simulink model "MOTHERofALL3"  (Simulink 7.7)
settings: Solver=VariableStepDiscrete  StartTime=0  StopTime=2  RelTol=1e-3
undefined symbols (not defined in the file): Acid, Lead, Ptotal, Qtotal, ts
libraries: powerlib x20, powerlib_extras x7, simulink x5, electricdrivelib x1
settings Model: Creator=chico  LastModifiedBy=elacpr

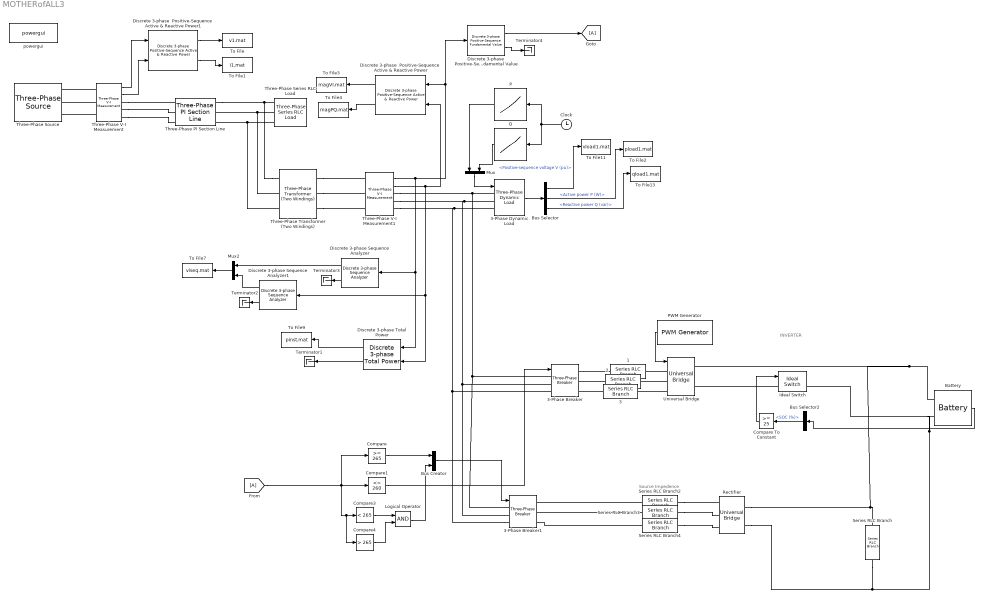
== system MOTHERofALL3 ==
  note: Source Impedence
  note: INVERTER
  1 : powerlib/Elements/Series RLC Branch  PhysicalDomain=powersysdomain  SubClassName=unknown  LeftPortType=p1  RightPortType=p1  LConnTagsString=__new0  RConnTagsString=__new0  BranchType=L  Resistance=1  Inductance=1  SetiL0=off  InitialCurrent=0  Capacitance=1e-6  Setx0=off  InitialVoltage=0  Measurements=None
  2 : powerlib/Elements/Series RLC Branch  PhysicalDomain=powersysdomain  SubClassName=unknown  LeftPortType=p1  RightPortType=p1  LConnTagsString=__new0  RConnTagsString=__new0  BranchType=L  Resistance=1  Inductance=1  SetiL0=off  InitialCurrent=0  Capacitance=1e-6  Setx0=off  InitialVoltage=0  Measurements=None
  3 : powerlib/Elements/Series RLC Branch  PhysicalDomain=powersysdomain  SubClassName=unknown  LeftPortType=p1  RightPortType=p1  LConnTagsString=__new0  RConnTagsString=__new0  BranchType=L  Resistance=1  Inductance=1  SetiL0=off  InitialCurrent=0  Capacitance=1e-6  Setx0=off  InitialVoltage=0  Measurements=None
  3-Phase Dynamic Load : powerlib/Elements/Three-Phase Dynamic Load  SystemSampleTime=-1  NominalVoltage=[ 400 60 ]  ActiveReactivePowers=[50 25]  PositiveSequence=[0.292838 -10.4312]  ExternalControl=on  NpNq="[1  1]"  TimeConstants="[0  0  0  0]"  MinimumVoltage=0.7  LoadFlowParameters=[4 50 0 0 25]
  3-Phase Breaker : powerlib/Elements/Three-Phase Breaker  SystemSampleTime=-1  InitialState=open  SwitchA=on  SwitchB=on  SwitchC=on  SwitchTimes="[4/60  10/60]"  External=on  BreakerResistance=0.001  SnubberResistance=1e6  SnubberCapacitance=inf  Measurements=None
  3-Phase Breaker1 : powerlib/Elements/Three-Phase Breaker  SystemSampleTime=-1  InitialState=open  SwitchA=on  SwitchB=on  SwitchC=on  SwitchTimes="[4/60  10/60]"  External=on  BreakerResistance=0.001  SnubberResistance=1e6  SnubberCapacitance=inf  Measurements=None
  Battery : electricdrivelib/Extra Sources/Battery  SystemSampleTime=-1  BatType=Lead-Acid  ShowDetailedParameters=off  NomV=240  NomQ=10  SOC=80  PresetModel=off  MaxQ=1.6154  FullV=1.4136  Dis_rate=0.3  R=0.008  Normal_OP=1.4423  expZone="[1.3017         0.3]"  Dis_Char=off  current=[1.5 3]  Units=Ampere-hour  Batt_Tr=30
  Bus Creator : BusCreator  Inputs=2
  Bus Selector : BusSelector  OutputSignals=Positive-sequence voltage V (pu),Active power P (W),Reactive power Q (var)
  Bus Selector2 : BusSelector  OutputSignals=SOC (%)
  Clock : Clock
  Compare : simulink/Logic and Bit Operations/Compare To Constant  SystemSampleTime=-1  relop=>=  const=265  LogicOutDataTypeMode=uint8
  Compare To Constant : simulink/Logic and Bit Operations/Compare To Constant  SystemSampleTime=-1  relop=>=  const=25  LogicOutDataTypeMode=uint8
  Compare1 : simulink/Logic and Bit Operations/Compare To Constant  SystemSampleTime=-1  relop=<=  const=260  LogicOutDataTypeMode=uint8
  Compare3 : simulink/Logic and Bit Operations/Compare To Constant  SystemSampleTime=-1  relop=<  const=265  LogicOutDataTypeMode=uint8
  Compare4 : simulink/Logic and Bit Operations/Compare To Constant  SystemSampleTime=-1  relop=>  const=265  LogicOutDataTypeMode=uint8
  Discrete 3-phase Positive-Sequence Fundamental Value : powerlib_extras/Discrete Measurements/Discrete 3-phase Positive-Sequence Fundamental Value  SystemSampleTime=-1  Freq=60  Par_Init=[0 0]  Ts=50e-6
  Discrete 3-phase Sequence Analyzer : powerlib_extras/Discrete Measurements/Discrete 3-phase Sequence Analyzer  SystemSampleTime=-1  Freq=60  n=1  seq=Positive  Par_Init=[0 0]  Ts=50e-6
  Discrete 3-phase Sequence Analyzer1 : powerlib_extras/Discrete Measurements/Discrete 3-phase Sequence Analyzer  SystemSampleTime=-1  Freq=60  n=1  seq=Positive  Par_Init=[0 0]  Ts=50e-6
  Discrete 3-phase Total Power : powerlib_extras/Discrete Measurements/Discrete 3-phase Total Power  SystemSampleTime=-1  Freq=60  Par_Vinit=[0 0]  Par_Iinit=[0 0]  Ts=50e-6
  Discrete 3-phase  Positive-Sequence  Active & Reactive Power : powerlib_extras/Discrete Measurements/Discrete 3-phase  Positive-Sequence  Active & Reactive Power  SystemSampleTime=-1  Freq=60  Par_Vinit=[0 0]  Par_Iinit=[0 0]  Ts=50e-6
  Discrete 3-phase  Positive-Sequence  Active & Reactive Power1 : powerlib_extras/Discrete Measurements/Discrete 3-phase  Positive-Sequence  Active & Reactive Power  SystemSampleTime=-1  Freq=60  Par_Vinit=[0 0]  Par_Iinit=[0 0]  Ts=50e-6
  Ideal Switch : powerlib/Power Electronics/Ideal Switch  SystemSampleTime=-1  Ron=0.001  Lon=0  IC=0  Rs=1e5  Cs=inf  Measurements=on
  Logical Operator : Logic  AllPortsSameDT=off  OutDataTypeStr=boolean
  Mux : Mux  Inputs=2
  Mux2 : Mux  Inputs=2
  P : Lookup  InputValues=ts  Table=Ptotal
  PWM Generator : powerlib_extras/Control  Blocks/PWM Generator  SystemSampleTime=-1  GeneratorMode="3-arm  bridge (6 pulses)"  Fc=1080  Internal=on  mIndex=0.4  Freq=50  Phase=0
  Q : Lookup  InputValues=ts  Table=Qtotal
  Rectifier : powerlib/Power Electronics/Universal Bridge  SystemSampleTime=-1  Arms=3  SnubberResistance=100  SnubberCapacitance=0.1e-6  Device=Diodes  Ron=1e-3  Lon=0  ForwardVoltages="[  0.8  0.8  ]"  ForwardVoltage=.8  GTOparameters=[ 10e-6 , 20e-6 ]  IGBTparameters=[ 1e-6 , 2e-6 ]  Measurements=Device currents  Measurements_2=None  converterType=Rectifier
  Series RLC Branch : powerlib/Elements/Series RLC Branch  PhysicalDomain=powersysdomain  SubClassName=unknown  LeftPortType=p1  RightPortType=p1  LConnTagsString=__new0  RConnTagsString=__new0  BranchType=C  Resistance=5  Inductance=1e-3  SetiL0=off  InitialCurrent=0  Capacitance=470e-6  Setx0=off  InitialVoltage=0  Measurements=None
  Series RLC Branch2 : powerlib/Elements/Series RLC Branch  PhysicalDomain=powersysdomain  SubClassName=unknown  LeftPortType=p1  RightPortType=p1  LConnTagsString=__new0  RConnTagsString=__new0  BranchType=RL  Resistance=0.5  Inductance=1e-3  SetiL0=off  InitialCurrent=0  Capacitance=200e-6  Setx0=off  InitialVoltage=0  Measurements=None
  Series RLC Branch3 : powerlib/Elements/Series RLC Branch  PhysicalDomain=powersysdomain  SubClassName=unknown  LeftPortType=p1  RightPortType=p1  LConnTagsString=__new0  RConnTagsString=__new0  BranchType=RL  Resistance=0.5  Inductance=1e-3  SetiL0=off  InitialCurrent=0  Capacitance=200e-6  Setx0=off  InitialVoltage=0  Measurements=None
  Series RLC Branch4 : powerlib/Elements/Series RLC Branch  PhysicalDomain=powersysdomain  SubClassName=unknown  LeftPortType=p1  RightPortType=p1  LConnTagsString=__new0  RConnTagsString=__new0  BranchType=RL  Resistance=0.5  Inductance=1e-3  SetiL0=off  InitialCurrent=0  Capacitance=200e-6  Setx0=off  InitialVoltage=0  Measurements=None
  Terminator{1..4} (4 alike) : Terminator
  Three-Phase PI Section Line : powerlib/Elements/Three-Phase PI Section Line  PhysicalDomain=powersysdomain  SubClassName=unknown  LeftPortType=p1  RightPortType=p1  LConnTagsString=a|b|c  RConnTagsString=A|B|C  Frequency=60  Resistances=[ 0.01273 0.3864]  Inductances="[ 0.9337e-3  4.1264e-3]"  Capacitances=[12.74e-9 7.751e-9]  Length=10
  Three-Phase Series RLC Load : powerlib/Elements/Three-Phase Series RLC Load  PhysicalDomain=powersysdomain  SubClassName=unknown  LeftPortType=p1  RightPortType=p1  LConnTagsString=A|B|C  Configuration=Y (grounded)  NominalVoltage=13800  NominalFrequency=60  ActivePower=10e6  InductivePower=1000  CapacitivePower=0  Measurements=None  LoadType=constant Z
  Three-Phase Transformer (Two Windings) : powerlib/Elements/Three-Phase Transformer (Two Windings)  SystemSampleTime=-1  Winding1Connection=Yg  UNITS=SI  NominalPower=[ 25e3 , 60 ]  Winding1=[13800 27.648 0.220022]  Winding2Connection=Yg  Winding2=[240 0.00384 0]  SetSaturation=off  Rm=1.3824e5  Lm=366  Saturation=[0 0;6.6653e-005 1910.3;0.027772 2419.7]  Hysteresis=off  DataFile='hysteresis'  SetInitialFlux=off  InitialFluxes=[1273.5 -1273.5 1114.3]  Measurements=None  MoreParameters=off  BreakLoop=off  DataType=on  TransfoNumber=1
  Three-Phase V-I Measurement : powerlib/Measurements/Three-Phase V-I Measurement  SystemSampleTime=-1  VoltageMeasurement=phase-to-ground  SetLabelV=off  LabelV=Vabc  Vpu=off  VpuLL=off  CurrentMeasurement=yes  SetLabelI=off  LabelI=Iabc  Ipu=off  Pbase=100e6  Vbase=500e3  OutputType=Complex  PhasorSimulation=off  PSBequivalent=0
  Three-Phase V-I Measurement1 : powerlib/Measurements/Three-Phase V-I Measurement  SystemSampleTime=-1  VoltageMeasurement=phase-to-phase  SetLabelV=off  LabelV=Vabc  Vpu=off  VpuLL=off  CurrentMeasurement=yes  SetLabelI=off  LabelI=Iabc  Ipu=off  Pbase=100e6  Vbase=240  OutputType=Complex  PhasorSimulation=off  PSBequivalent=0
  Three-Phase Source : powerlib/Electrical Sources/Three-Phase Source  SystemSampleTime=-1  Voltage=13800  PhaseAngle=0  Frequency=60  InternalConnection=Yg  SpecifyImpedance=off  Resistance=0.001  Inductance=0.000001  ShortCircuitLevel=100e6  BaseVoltage=25e3  XRratio=7  BusType=swing  Pref=0  Qref=0  Qmin=-inf  Qmax=inf
  To File : ToFile  Filename=v1.mat  MatrixName=v1
      settings: Decimation=200
  To File1 : ToFile  Filename=i1.mat  MatrixName=i1
      settings: Decimation=200
  To File11 : ToFile  Filename=vload1.mat  MatrixName=vl1
      settings: Decimation=20000
  To File13 : ToFile  Filename=qload1.mat  MatrixName=ql1
      settings: Decimation=20000
  To File2 : ToFile  Filename=pload1.mat  MatrixName=pl1
      settings: Decimation=20000
  To File3 : ToFile  Filename=magVI.mat  MatrixName=vi
      settings: Decimation=20000
  To File4 : ToFile  Filename=magPQ.mat  MatrixName=pq
      settings: Decimation=20000
  To File7 : ToFile  Filename=viseq.mat  MatrixName=viseq
      settings: Decimation=20000
  To File9 : ToFile  Filename=pinst.mat  MatrixName=pinst
      settings: Decimation=200
  Universal Bridge : powerlib/Power Electronics/Universal Bridge  SystemSampleTime=-1  Arms=3  SnubberResistance=1e5  SnubberCapacitance=inf  Device=IGBT / Diodes  Ron=1e-3  Lon=0  ForwardVoltages="[  0  0  ]"  ForwardVoltage=0  GTOparameters=[ 10e-6 , 20e-6 ]  IGBTparameters=[ 1e-6 , 2e-6 ]  Measurements=None  Measurements_2=None  converterType=Rectifier
  powergui : powerlib/powergui  Priority=1  SystemSampleTime=-1  SimulationMode=Discrete  SampleTime=50e-4  frequency=60  SPID=off  DisableSnubberDevices=off  DisableRonSwitches=off  DisableVfSwitches=off  SwTol=0  Interpol=off  DisplayEquations=off  FunctionMessages=off  frequencyindice=60  Pbase=100e6  ErrMax=1e-4  Iterations=50  UnitsV=kV  UnitsW=MW  echomessages=off  HookPort=off  EnableUseOfTLC=off  x0status=blocks  RestoreLinks=warning  ResistiveCurrentMeasurement=off  Ylog=off  Xlog=on  ShowGrid=off  save=off  variable=ZData  ZoomFFT=off  StartTime=0.0  cycles=1  DisplayStyle=1  FreqAxis=off  MaxFrequency=1000  frequencyindicesteady=1  display=off  methode=off
  wires:
  P/1 -> Mux/1
  Q/1 -> Mux/2
  Clock/1 -> Q/1, P/1
  Mux/1 -> 3-Phase Dynamic Load/1
  Three-Phase V-I Measurement1/1 -> Discrete 3-phase Total Power/1, Discrete 3-phase Sequence Analyzer/1, Discrete 3-phase  Positive-Sequence  Active & Reactive Power/1, Discrete 3-phase Positive-Sequence Fundamental Value/1
  Three-Phase V-I Measurement1/2 -> Discrete 3-phase Total Power/2, Discrete 3-phase Sequence Analyzer1/1, Discrete 3-phase  Positive-Sequence  Active & Reactive Power/2
  Discrete 3-phase  Positive-Sequence  Active & Reactive Power/2 -> To File4/1
  Discrete 3-phase Sequence Analyzer/1 -> Mux2/1
  Discrete 3-phase Sequence Analyzer1/1 -> Mux2/2
  Mux2/1 -> To File7/1
  Discrete 3-phase Total Power/1 -> To File9/1
  Discrete 3-phase Total Power/2 -> Terminator1/1
  Discrete 3-phase Sequence Analyzer1/2 -> Terminator2/1
  Discrete 3-phase Sequence Analyzer/2 -> Terminator3/1
  3-Phase Dynamic Load/1 -> Bus Selector/1
  Bus Selector/1 -> To File11/1  "<Positive-sequence voltage V (pu)>"
  Bus Selector/2 -> To File2/1  "<Active power P (W)>"
  Bus Selector/3 -> To File13/1  "<Reactive power Q (var)>"
  Three-Phase V-I Measurement/1 -> Discrete 3-phase  Positive-Sequence  Active & Reactive Power1/1
  Three-Phase V-I Measurement/2 -> Discrete 3-phase  Positive-Sequence  Active & Reactive Power1/2
  Discrete 3-phase  Positive-Sequence  Active & Reactive Power1/1 -> To File/1
  Discrete 3-phase  Positive-Sequence  Active & Reactive Power1/2 -> To File1/1
  Compare3/1 -> Logical Operator/1
  Compare4/1 -> Logical Operator/2
  PWM Generator/1 -> Universal Bridge/1
  Bus Selector2/1 -> Compare To Constant/1  "<SOC (%)>"
  Compare To Constant/1 -> Ideal Switch/1
  Compare1/1 -> 3-Phase Breaker/1
  Compare/1 -> Bus Creator/1
  Logical Operator/1 -> Bus Creator/2
  Bus Creator/1 -> 3-Phase Breaker1/1
  Battery/1 -> Bus Selector2/1
  [A] -> Compare/1, Compare1/1, Compare3/1, Compare4/1
  Discrete 3-phase  Positive-Sequence  Active & Reactive Power/1 -> To File3/1
  Discrete 3-phase Positive-Sequence Fundamental Value/2 -> Terminator4/1
  Discrete 3-phase Positive-Sequence Fundamental Value/1 -> [A]
  connections:
  Three-Phase V-I Measurement/LConn3 -- Three-Phase Source/RConn3
  Three-Phase V-I Measurement/LConn2 -- Three-Phase Source/RConn2
  Three-Phase V-I Measurement/LConn1 -- Three-Phase Source/RConn1
  Three-Phase V-I Measurement/RConn1 -- Three-Phase PI Section Line/LConn1
  Three-Phase V-I Measurement/RConn2 -- Three-Phase PI Section Line/LConn2
  Three-Phase V-I Measurement/RConn3 -- Three-Phase PI Section Line/LConn3
  Three-Phase Transformer (Two Windings)/LConn1 -- Three-Phase PI Section Line/RConn1 -- Three-Phase Series RLC Load/LConn1
  Three-Phase Series RLC Load/LConn2 -- Three-Phase PI Section Line/RConn2 -- Three-Phase Transformer (Two Windings)/LConn2
  Three-Phase Series RLC Load/LConn3 -- Three-Phase PI Section Line/RConn3 -- Three-Phase Transformer (Two Windings)/LConn3
  Three-Phase Transformer (Two Windings)/RConn3 -- Three-Phase V-I Measurement1/LConn3
  Three-Phase Transformer (Two Windings)/RConn2 -- Three-Phase V-I Measurement1/LConn2
  Three-Phase Transformer (Two Windings)/RConn1 -- Three-Phase V-I Measurement1/LConn1
  Series RLC Branch2/RConn1 -- 3-Phase Breaker1/RConn1
  Series RLC Branch3/RConn1 -- 3-Phase Breaker1/RConn2
  Series RLC Branch4/RConn1 -- 3-Phase Breaker1/RConn3
  3-Phase Breaker1/LConn1 -- 3-Phase Breaker/LConn1 -- Three-Phase V-I Measurement1/RConn1 -- 3-Phase Dynamic Load/LConn1
  Rectifier/RConn1 -- Battery/LConn1 -- Universal Bridge/RConn1 -- Series RLC Branch/LConn1
  Rectifier/RConn2 -- Battery/LConn2 -- Ideal Switch/RConn1 -- Series RLC Branch/RConn1
  Universal Bridge/LConn1 -- 1/LConn1
  Universal Bridge/LConn2 -- 2/LConn1
  Universal Bridge/LConn3 -- 3/LConn1
  Ideal Switch/LConn1 -- Universal Bridge/RConn2
  2/RConn1 -- 3-Phase Breaker/RConn2
  3/RConn1 -- 3-Phase Breaker/RConn3
  Series RLC Branch2/LConn1 -- Rectifier/LConn1
  Series RLC Branch3/LConn1 -- Rectifier/LConn2
  Series RLC Branch4/LConn1 -- Rectifier/LConn3
  3-Phase Breaker1/LConn3 -- 3-Phase Breaker/LConn3 -- Three-Phase V-I Measurement1/RConn3 -- 3-Phase Dynamic Load/LConn3
  3-Phase Breaker1/LConn2 -- 3-Phase Breaker/LConn2 -- Three-Phase V-I Measurement1/RConn2 -- 3-Phase Dynamic Load/LConn2
  1/RConn1 -- 3-Phase Breaker/RConn1
